simulink model "model"  (R2018b)
settings: Solver=VariableStepAuto  StartTime=0.0  StopTime=10.0  RelTol=1e-3
values from neighbouring files (symbols this model uses):
  dt = 1/10    (= 0.1)    [runScript.m]
undefined symbols (not defined in the file or in its folder): Vx, Vx_prev, Vy, Vy_prev, Vz, Vz_prev
settings Model: Creator=Leshi  LastModifiedBy=Leshi

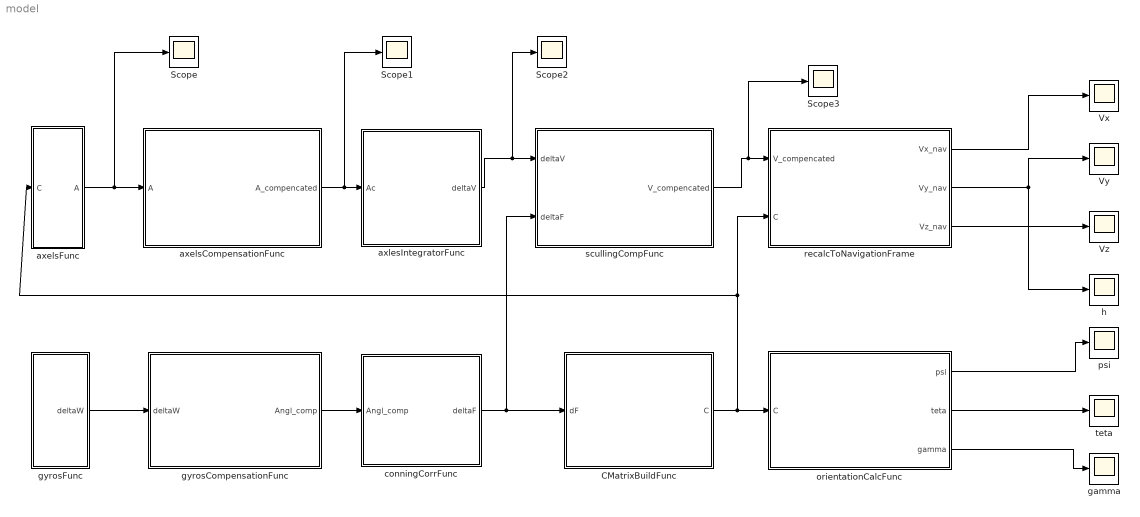
== system model ==
  CMatrixBuildFunc : MATLAB Function  TreatAsAtomicUnit=on
  Scope{,1..3} (4 alike) : Scope
  Vx : Scope
  Vy : Scope
  Vz : Scope
  axelsCompensationFunc : MATLAB Function  TreatAsAtomicUnit=on
  axelsFunc : MATLAB Function  TreatAsAtomicUnit=on
  axlesIntegratorFunc : MATLAB Function  TreatAsAtomicUnit=on
  conningCorrFunc : MATLAB Function  TreatAsAtomicUnit=on
  gamma : Scope
  gyrosCompensationFunc : MATLAB Function  TreatAsAtomicUnit=on
  gyrosFunc : MATLAB Function  TreatAsAtomicUnit=on
  h : Scope
  orientationCalcFunc : MATLAB Function  TreatAsAtomicUnit=on
  psi : Scope
  recalcToNavigationFrame : MATLAB Function  TreatAsAtomicUnit=on
  scullingCompFunc : MATLAB Function  TreatAsAtomicUnit=on
  teta : Scope
  wires:
  gyrosFunc/1(deltaW) -> gyrosCompensationFunc/1(deltaW)
  recalcToNavigationFrame/1(Vx_nav) -> Vx/1
  recalcToNavigationFrame/3(Vz_nav) -> Vz/1
  recalcToNavigationFrame/2(Vy_nav) -> h/1, Vy/1
  orientationCalcFunc/1(psi) -> psi/1
  orientationCalcFunc/2(teta) -> teta/1
  orientationCalcFunc/3(gamma) -> gamma/1
  gyrosCompensationFunc/1(Angl_comp) -> conningCorrFunc/1(Angl_comp)
  axlesIntegratorFunc/1(deltaV) -> Scope2/1, scullingCompFunc/1(deltaV)
  axelsFunc/1(A) -> Scope/1, axelsCompensationFunc/1(A)
  axelsCompensationFunc/1(A_compencated) -> Scope1/1, axlesIntegratorFunc/1(Ac)
  conningCorrFunc/1(deltaF) -> scullingCompFunc/2(deltaF), CMatrixBuildFunc/1(dF)
  scullingCompFunc/1(V_compencated) -> Scope3/1, recalcToNavigationFrame/1(V_compencated)
  CMatrixBuildFunc/1(C) -> axelsFunc/1(C), recalcToNavigationFrame/2(C), orientationCalcFunc/1(C)

== matlab function model/gyrosFunc ==
  data: deltaW output size=[1, 3]
% Give increment of anular vels
function deltaW = Gyros()

Wx = awgn(0,10,'measured');
Wy = awgn(0,10,'measured');
Wz = awgn(0,10,'measured');

deltaW = [Wx, Wy, Wz];

== matlab function model/axelsFunc ==
  data: C input size=[3, 3]; A output size=[1, 3]; g parameter
% Give pure aceleration
function A = Axels(C, g)

C_obrat = inv(C);
g_cur = g * C_obrat;

% Q_ = quatconj(Q);
% gCurrnet = Q * g * Q_;

Ax = awgn(real(g_cur(1)),10,'measured');
Ay = awgn(real(g_cur(2)),10,'measured');
Az = awgn(real(g_cur(3)),10,'measured');

A = [Ax, Ay, Az];

== matlab function model/axelsCompensationFunc ==
  data: A input size=[1, 3]; A_compencated output; g parameter size=[1, 3]
function A_compencated  = AxelsCompensation(A, g)
Ax_compencated = A(1);
Ay_compencated = A(2) - g(2);
Az_compencated = A(3);

A_compencated = [Ax_compencated, Ay_compencated, Az_compencated];

== matlab function model/gyrosCompensationFunc ==
  data: Angl_comp output size=[1, 3]; deltaW input size=[1, 3]
% Returns compencated increment of angulag vel
function Angl_comp = GyrosCompensation(deltaW)
Wx_c = deltaW(1);
Wy_c = deltaW(2);
Wz_c = deltaW(3);

Angl_comp= [Wx_c, Wy_c, Wz_c];

== matlab function model/scullingCompFunc ==
  data: deltaV input size=[1, 3]; deltaF input; V_compencated output size=[1, 3]; Vx parameter; Vy parameter; Vz parameter; Vx_prev parameter; Vy_prev parameter; Vz_prev parameter
function V_compencated = ScullingCompensation(deltaV, deltaF, Vx, Vy, Vz, Vx_prev, Vy_prev, Vz_prev)
Vx = Vx_prev + Vy_prev * deltaF(3) - Vz_prev * deltaF(2) + deltaV(1);
Vy = Vy_prev + Vz_prev * deltaF(1) - Vx_prev * deltaF(3) + deltaV(2);
Vz = Vz_prev + Vx_prev * deltaF(2) - Vy_prev * deltaF(1) + deltaV(3);

Vx_prev = Vx;
Vy_prev = Vy;
Vz_prev = Vz;

V_compencated = [Vx, Vy, Vz];

== matlab function model/recalcToNavigationFrame ==
  data: V_compencated input; C input size=[3, 3]; Vx_nav output; Vy_nav output; Vz_nav output
function [Vx_nav, Vy_nav, Vz_nav] = BodyToNavCalc(V_compencated, C)

% Q_ = quaternion(q0, -q1, -q2, -q3);
% V_nav = Q .* V_compencated .* Q_;

V_nav = V_compencated * C;

Vx_nav = V_nav(1);
Vy_nav = V_nav(2);
Vz_nav = V_nav(3);

% Vx_nav = V_compencated(1);
% Vy_nav = V_compencated(2);
% Vz_nav = V_compencated(3);

== matlab function model/CMatrixBuildFunc ==
  data: dF input size=[1, 3]; C_prev parameter size=[3, 3]; C output size=[3, 3]
function C  = QaternionBuild(dF, C_prev)

% size(C_prev)
% size(dF)

C = C_prev ;
% C_prev = C;

== matlab function model/conningCorrFunc ==
  data: deltaF output size=[1, 3]; Angl_comp input size=[1, 3]
% Returns compencated increment of angulag vel
function deltaF  = ConingCorrection(Angl_comp)
dFx = Angl_comp(1);
dFy = Angl_comp(2);
dFz = Angl_comp(3);

deltaF = [dFx dFy dFz];

== matlab function model/orientationCalcFunc ==
  data: psi output; C input size=[3,3]; teta output; gamma output
function [psi, teta, gamma] = OrientationAnglesCalc(C)
teta = atan2(real(C(3, 2)), sqrt(real(C(3,1)^2 + real(C(3, 3)^2))));
psi = atan2(real(C(1,2)), real(C(2,2)));
gamma = - atan2(real(C(3, 1)), real(C(3, 3)));
% 
% [q0, q1, q2, q3] = parts(Q);
% 
% psi = atan2(- (2 * q1 * q3  - 2 * q0 * q2), (2 * q1^2  + 2 * q0^2 - 1)));
% teta = asin(2 * q1 * q2  + 2 * q0 * q3);
% gamma = atan2( - (2 * q2 * q3 - 2 * q0 * q1), (2 * q0^2 + 2 * q2^2 - 1)));

== matlab function model/axlesIntegratorFunc ==
  data: Ac input size=[1, 3]; deltaV output size=[1, 3]; dt parameter; Vx_prev parameter; Vy_prev parameter; Vz_prev parameter
function deltaV = AIntegrator(Ac, dt, Vx_prev, Vy_prev, Vz_prev)
coder.extrinsic('assignin');

Vx = Vx_prev + Ac(1) * dt;
Vy = Vy_prev + Ac(2) * dt;
Vz = Vz_prev + Ac(3) * dt;

assignin('base', 'Vx_prev', Vx);
assignin('base', 'Vy_prev', Vy);
assignin('base', 'Vz_prev', Vz);

deltaV = [Vx, Vy, Vz];
